simulink model "fft_biplex_test3"  (Simulink 7.6)
settings: Solver=ode45  StartTime=0.0  StopTime=5000  RelTol=1e-3
libraries: xbsIndex_r4 x1382, casper_library x82, monroe_library x27, xps_library x17, dspsigops x16, simulink x1
(part 9 of 13)

== system fft_biplex_test3/fft_biplex_real_4x1/biplex_core/fft_stage_2/delay_f ==
  In1 : Inport
  Constant2 : xbsIndex_r4/Constant  arith_type=Boolean  const=1  n_bits=1  bin_pt=0  explicit_period=on  period=1  equ=P=C  opselect=C  inp2=PCIN>>17  opr=+  inp1=P  carry=CIN  dbl_ovrd=off  block_type=constant
      settings: block_version=9.1.01
  Counter : xbsIndex_r4/Counter  cnt_type=Count Limited  cnt_to=DelayLen - bram_latency - 1  operation=Up  start_count=0  cnt_by_val=1  arith_type=Unsigned  n_bits=BitWidth  bin_pt=0  load_pin=off  rst=off  en=off  explicit_period=on  period=1  dbl_ovrd=off  use_behavioral_HDL=off  implementation=Fabric  use_rpm=off  block_type=counter
      settings: xl_area=[0, 0, 0, 0, 0, 0, 0]  block_version=9.1.01
  Single Port RAM : xbsIndex_r4/Single Port RAM  depth=2^BitWidth  initVector=0  distributed_mem=Block RAM  write_mode=Read Before Write  rst=off  init_reg=0  en=off  latency=bram_latency  dbl_ovrd=off  optimize=Area  use_rpm=off  block_type=spram
      settings: xl_area=[0, 0, 0, 0, 0, 0, 0]  block_version=9.1.01
  Out1 : Outport
  wires:
  Single Port RAM/1 -> Out1/1
  Counter/1 -> Single Port RAM/1
  In1/1 -> Single Port RAM/2
  Constant2/1 -> Single Port RAM/3

== system fft_biplex_test3/fft_biplex_real_4x1/biplex_core/fft_stage_3/butterfly_direct ==
  a : Inport
  b : Inport  Port=2
  sync : Inport  Port=3
  shift : Inport  Port=4
  Delay : xbsIndex_r4/Delay  en=off  latency=add_latency + 1  dbl_ovrd=off  reg_retiming=off  block_type=delay
      settings: xl_area=[0, 0, 0, 0, 0, 0, 0]  block_version=9.1.01
  Logical : xbsIndex_r4/Logical  logical_function=OR  inputs=4  en=off  latency=0  precision=Full  arith_type=Unsigned  n_bits=16  bin_pt=0  align_bp=on  dbl_ovrd=off  block_type=logical
      settings: block_version=10.1.1
  Register{,1..5} (6 alike) : xbsIndex_r4/Register  init=0  rst=off  en=off  dbl_ovrd=off  block_type=register
      settings: block_version=11.4
  Scale{,1..3} (4 alike) : xbsIndex_r4/Scale  scale_factor=-shift  dbl_ovrd=off  block_type=scale
      settings: block_version=9.1.01
  Terminator : Terminator
  convert_of1 : Subsystem  AncestorBlock=casper_library/Misc/convert_of  mask(convert_of){bit_width_i=24, binary_point_i=19, bit_width_o=18, binary_point_o=17, latency=1, overflow=Wrap, quantization=Truncate}
      mask prompts: bit_width_i "Bit Width In"; binary_point_i "Binary Point In"; bit_width_o "Bit Width Out"; binary_point_o "Binary Point Out"; overflow "Overflow Behaviour"; quantization "Quantization Behaviour"
      mask help:
      | Converts from one 2's complement bit-width
      | and/or binary point position to another.
      | Includes underflow/overflow indicator.
      mask init: same as fft_biplex_test3/fft_biplex_real_4x1/biplex_core/fft_stage_1/butterfly_direct/convert_of1
      settings: AttributesFormatString=[24,19]->[18,17]
      mask StyleString: edit,edit,edit,edit,edit,popup(Wrap|Saturate|Error),popup(Truncate|Round  (unbiased: +/- Inf)|Round  (unbiased: even values))
  convert_of2 : Subsystem  AncestorBlock=casper_library/FFTs/butterfly_direct/convert_of1  mask(convert_of){bit_width_i=24, binary_point_i=19, bit_width_o=18, binary_point_o=17, latency=1, overflow=Wrap, quantization=Truncate}
      mask prompts: bit_width_i "Bit Width In"; binary_point_i "Binary Point In"; bit_width_o "Bit Width Out"; binary_point_o "Binary Point Out"; overflow "Overflow Behaviour"; quantization "Quantization Behaviour"
      mask help:
      | Converts from one 2's complement bit-width
      | and/or binary point position to another.
      | Includes underflow/overflow indicator.
      mask init: same as fft_biplex_test3/fft_biplex_real_4x1/biplex_core/fft_stage_1/butterfly_direct/convert_of1
      settings: AttributesFormatString=[24,19]->[18,17]
      mask StyleString: edit,edit,edit,edit,edit,popup(Wrap|Saturate|Error),popup(Truncate|Round  (unbiased: +/- Inf)|Round  (unbiased: even values))
  convert_of3 : Subsystem  AncestorBlock=casper_library/FFTs/butterfly_direct/convert_of1  mask(convert_of){bit_width_i=24, binary_point_i=19, bit_width_o=18, binary_point_o=17, latency=1, overflow=Wrap, quantization=Truncate}
      mask prompts: bit_width_i "Bit Width In"; binary_point_i "Binary Point In"; bit_width_o "Bit Width Out"; binary_point_o "Binary Point Out"; overflow "Overflow Behaviour"; quantization "Quantization Behaviour"
      mask help:
      | Converts from one 2's complement bit-width
      | and/or binary point position to another.
      | Includes underflow/overflow indicator.
      mask init: same as fft_biplex_test3/fft_biplex_real_4x1/biplex_core/fft_stage_1/butterfly_direct/convert_of1
      settings: AttributesFormatString=[24,19]->[18,17]
      mask StyleString: edit,edit,edit,edit,edit,popup(Wrap|Saturate|Error),popup(Truncate|Round  (unbiased: +/- Inf)|Round  (unbiased: even values))
  convert_of4 : Subsystem  AncestorBlock=casper_library/FFTs/butterfly_direct/convert_of1  mask(convert_of){bit_width_i=24, binary_point_i=19, bit_width_o=18, binary_point_o=17, latency=1, overflow=Wrap, quantization=Truncate}
      mask prompts: bit_width_i "Bit Width In"; binary_point_i "Binary Point In"; bit_width_o "Bit Width Out"; binary_point_o "Binary Point Out"; overflow "Overflow Behaviour"; quantization "Quantization Behaviour"
      mask help:
      | Converts from one 2's complement bit-width
      | and/or binary point position to another.
      | Includes underflow/overflow indicator.
      mask init: same as fft_biplex_test3/fft_biplex_real_4x1/biplex_core/fft_stage_1/butterfly_direct/convert_of1
      settings: AttributesFormatString=[24,19]->[18,17]
      mask StyleString: edit,edit,edit,edit,edit,popup(Wrap|Saturate|Error),popup(Truncate|Round  (unbiased: +/- Inf)|Round  (unbiased: even values))
  dsp48_complex_add : Subsystem  mask{a_bit_width=18, a_bin_pt=17, bw_bit_width=input_bit_width+coeff_bit_width+1, bw_bin_pt=(input_bit_width - 1) + (coeff_bit_width-1)}
      mask prompts: a_bit_width "'a' bit width"; a_bin_pt "'a' binary point"; bw_bit_width "'bw' bit width"; bw_bin_pt "'bw' binary point"
  ri_to_c : casper_library/Misc/ri_to_c  SystemSampleTime=-1
  ri_to_c1 : casper_library/Misc/ri_to_c  SystemSampleTime=-1
  twiddle : Subsystem  AncestorBlock=casper_library/FFTs/Twiddle/twiddle_general_dsp48  mask(twiddle_general_dsp48){Coeffs=getfield( getfield( get_param( gcb,'UserData' ), 'parameters'),'Coeffs'), StepPeriod=2, coeffs_bram=off, coeff_bit_width=18, input_bit_width=18, add_latency=2, mult_latency=3, bram_latency=3, arch=Virtex5, use_hdl=on, use_embedded=off, quantization=Truncate, overflow=Wrap}
      mask prompts: Coeffs "Coefficients:"; StepPeriod "Coefficient Step Period (2^?)"; coeffs_bram "Store coefficients in BRAM"; coeff_bit_width "Coefficient Bit Width"; input_bit_width "Input Bit Width"; add_latency "Add Latency"; mult_latency "Mult Latency"; bram_latency "BRAM Latency"; arch "Architecture"; use_hdl "Use behavioural HDL for multipliers"; use_embedded "Use embedded multipliers"; quantization "Quantization Behavior"; overflow "Overflow Behavior"
      mask help:
      | Used in biplex pipelined FFT. Implements
      | (a+bi)(c+di) as (ac-bd)+i(ad+bc) with four
      | multipliers, manually instantiating dsp48 slices
      mask init:
      | twiddle_general_dsp48_init(gcb, ...
      |     'Coeffs', Coeffs, ...
      |     'StepPeriod', StepPeriod, ...
      |     'coeffs_bram', coeffs_bram, ...
      |     'coeff_bit_width', coeff_bit_width, ...
      |     'input_bit_width', input_bit_width, ...
      |     'add_latency', add_latency, ...
      |     'mult_latency', mult_latency, ...
      |     'bram_latency', bram_latency, ...
      |     'arch', arch, ...
      |     'use_hdl', use_hdl, ...
      |     'use_embedded', use_embedded, ...
      |     'quantization', quantization, ...
      |     'overflow', overflow)
      settings: AttributesFormatString=|
      | arch=Virtex5,
      |  input_bit_width=18,
      |  coeff_bit_width=18
      mask StyleString: edit,edit,checkbox,edit,edit,edit,edit,edit,popup(Virtex2Pro|Virtex5),checkbox,checkbox,popup(Truncate|Round  (unbiased: +/- Inf)|Round  (unbiased: Even Values)),popup(Wrap|Saturate|Error)
      mask CallbackString:
      | |||||||||use_hdl = get_param(gcb,'use_hdl');
      | visibs = get_param(gcb, 'MaskVisibilities');
      | if( strcmp(use_hdl,'on')),
      |     set_param(gcb, 'use_embedded','off');
      |     visibs{11} = 'off';
      | else,
      |     visibs{11} = 'on';
      | end
      | set_param(gcb, 'MaskVisibilities', visibs);|||
  a+bw : Outport
  a-bw : Outport  Port=2
  of : Outport  Port=3
  sync_out : Outport  Port=4
  wires:
  Register5/1 -> twiddle/1(a)
  Register4/1 -> twiddle/2(b)
  Register3/1 -> twiddle/3(sync)
  Register2/1 -> sync_out/1
  Register1/1 -> a-bw/1
  Register/1 -> a+bw/1
  dsp48_complex_add/4(a-bw_im) -> Scale3/1
  Logical/1 -> of/1
  shift/1 -> Terminator/1
  dsp48_complex_add/1(a+bw_re) -> Scale/1
  Delay/1 -> Register2/1
  ri_to_c1/1 -> Register1/1
  ri_to_c/1 -> Register/1
  a/1 -> Register5/1
  b/1 -> Register4/1
  sync/1 -> Register3/1
  twiddle/1(a_re) -> dsp48_complex_add/1(a_re)
  twiddle/2(a_im) -> dsp48_complex_add/2(a_im)
  twiddle/3(bw_re) -> dsp48_complex_add/3(bw_re)
  twiddle/4(bw_im) -> dsp48_complex_add/4(bw_im)
  twiddle/5(sync_out) -> Delay/1
  Scale/1 -> convert_of1/1(din)
  convert_of1/1(dout) -> ri_to_c/1
  dsp48_complex_add/2(a+bw_im) -> Scale1/1
  Scale1/1 -> convert_of2/1(din)
  convert_of2/1(dout) -> ri_to_c/2
  dsp48_complex_add/3(a-bw_re) -> Scale2/1
  Scale2/1 -> convert_of3/1(din)
  convert_of3/1(dout) -> ri_to_c1/1
  Scale3/1 -> convert_of4/1(din)
  convert_of4/1(dout) -> ri_to_c1/2
  convert_of1/2(of) -> Logical/1
  convert_of2/2(of) -> Logical/2
  convert_of3/2(of) -> Logical/3
  convert_of4/2(of) -> Logical/4

== system fft_biplex_test3/fft_biplex_real_4x1/biplex_core/fft_stage_3/delay_b ==
  In1 : Inport
  delay_slr : xbsIndex_r4/Delay  en=off  latency=DelayLen  dbl_ovrd=off  reg_retiming=off  block_type=delay
      settings: xl_area=[0, 0, 0, 0, 0, 0, 0]  block_version=9.1.01
  Out1 : Outport
  wires:
  In1/1 -> delay_slr/1
  delay_slr/1 -> Out1/1

== system fft_biplex_test3/fft_biplex_real_4x1/biplex_core/fft_stage_3/delay_f ==
  In1 : Inport
  delay_slr : xbsIndex_r4/Delay  en=off  latency=DelayLen  dbl_ovrd=off  reg_retiming=off  block_type=delay
      settings: xl_area=[0, 0, 0, 0, 0, 0, 0]  block_version=9.1.01
  Out1 : Outport
  wires:
  In1/1 -> delay_slr/1
  delay_slr/1 -> Out1/1

== system fft_biplex_test3/fft_biplex_real_4x1/biplex_core/fft_stage_4/butterfly_direct ==
  a : Inport
  b : Inport  Port=2
  sync : Inport  Port=3
  shift : Inport  Port=4
  Delay : xbsIndex_r4/Delay  en=off  latency=add_latency + 1  dbl_ovrd=off  reg_retiming=off  block_type=delay
      settings: xl_area=[0, 0, 0, 0, 0, 0, 0]  block_version=9.1.01
  Logical : xbsIndex_r4/Logical  logical_function=OR  inputs=4  en=off  latency=0  precision=Full  arith_type=Unsigned  n_bits=16  bin_pt=0  align_bp=on  dbl_ovrd=off  block_type=logical
      settings: block_version=10.1.1
  Register{,1..5} (6 alike) : xbsIndex_r4/Register  init=0  rst=off  en=off  dbl_ovrd=off  block_type=register
      settings: block_version=11.4
  Scale{,1..3} (4 alike) : xbsIndex_r4/Scale  scale_factor=-shift  dbl_ovrd=off  block_type=scale
      settings: block_version=9.1.01
  Terminator : Terminator
  convert_of1 : Subsystem  AncestorBlock=casper_library/Misc/convert_of  mask(convert_of){bit_width_i=24, binary_point_i=19, bit_width_o=18, binary_point_o=17, latency=1, overflow=Wrap, quantization=Truncate}
      mask prompts: bit_width_i "Bit Width In"; binary_point_i "Binary Point In"; bit_width_o "Bit Width Out"; binary_point_o "Binary Point Out"; overflow "Overflow Behaviour"; quantization "Quantization Behaviour"
      mask help:
      | Converts from one 2's complement bit-width
      | and/or binary point position to another.
      | Includes underflow/overflow indicator.
      mask init: same as fft_biplex_test3/fft_biplex_real_4x1/biplex_core/fft_stage_1/butterfly_direct/convert_of1
      settings: AttributesFormatString=[24,19]->[18,17]
      mask StyleString: edit,edit,edit,edit,edit,popup(Wrap|Saturate|Error),popup(Truncate|Round  (unbiased: +/- Inf)|Round  (unbiased: even values))
  convert_of2 : Subsystem  AncestorBlock=casper_library/FFTs/butterfly_direct/convert_of1  mask(convert_of){bit_width_i=24, binary_point_i=19, bit_width_o=18, binary_point_o=17, latency=1, overflow=Wrap, quantization=Truncate}
      mask prompts: bit_width_i "Bit Width In"; binary_point_i "Binary Point In"; bit_width_o "Bit Width Out"; binary_point_o "Binary Point Out"; overflow "Overflow Behaviour"; quantization "Quantization Behaviour"
      mask help:
      | Converts from one 2's complement bit-width
      | and/or binary point position to another.
      | Includes underflow/overflow indicator.
      mask init: same as fft_biplex_test3/fft_biplex_real_4x1/biplex_core/fft_stage_1/butterfly_direct/convert_of1
      settings: AttributesFormatString=[24,19]->[18,17]
      mask StyleString: edit,edit,edit,edit,edit,popup(Wrap|Saturate|Error),popup(Truncate|Round  (unbiased: +/- Inf)|Round  (unbiased: even values))
  convert_of3 : Subsystem  AncestorBlock=casper_library/FFTs/butterfly_direct/convert_of1  mask(convert_of){bit_width_i=24, binary_point_i=19, bit_width_o=18, binary_point_o=17, latency=1, overflow=Wrap, quantization=Truncate}
      mask prompts: bit_width_i "Bit Width In"; binary_point_i "Binary Point In"; bit_width_o "Bit Width Out"; binary_point_o "Binary Point Out"; overflow "Overflow Behaviour"; quantization "Quantization Behaviour"
      mask help:
      | Converts from one 2's complement bit-width
      | and/or binary point position to another.
      | Includes underflow/overflow indicator.
      mask init: same as fft_biplex_test3/fft_biplex_real_4x1/biplex_core/fft_stage_1/butterfly_direct/convert_of1
      settings: AttributesFormatString=[24,19]->[18,17]
      mask StyleString: edit,edit,edit,edit,edit,popup(Wrap|Saturate|Error),popup(Truncate|Round  (unbiased: +/- Inf)|Round  (unbiased: even values))
  convert_of4 : Subsystem  AncestorBlock=casper_library/FFTs/butterfly_direct/convert_of1  mask(convert_of){bit_width_i=24, binary_point_i=19, bit_width_o=18, binary_point_o=17, latency=1, overflow=Wrap, quantization=Truncate}
      mask prompts: bit_width_i "Bit Width In"; binary_point_i "Binary Point In"; bit_width_o "Bit Width Out"; binary_point_o "Binary Point Out"; overflow "Overflow Behaviour"; quantization "Quantization Behaviour"
      mask help:
      | Converts from one 2's complement bit-width
      | and/or binary point position to another.
      | Includes underflow/overflow indicator.
      mask init: same as fft_biplex_test3/fft_biplex_real_4x1/biplex_core/fft_stage_1/butterfly_direct/convert_of1
      settings: AttributesFormatString=[24,19]->[18,17]
      mask StyleString: edit,edit,edit,edit,edit,popup(Wrap|Saturate|Error),popup(Truncate|Round  (unbiased: +/- Inf)|Round  (unbiased: even values))
  dsp48_complex_add : Subsystem  mask{a_bit_width=18, a_bin_pt=17, bw_bit_width=input_bit_width+coeff_bit_width+1, bw_bin_pt=(input_bit_width - 1) + (coeff_bit_width-1)}
      mask prompts: a_bit_width "'a' bit width"; a_bin_pt "'a' binary point"; bw_bit_width "'bw' bit width"; bw_bin_pt "'bw' binary point"
  ri_to_c : casper_library/Misc/ri_to_c  SystemSampleTime=-1
  ri_to_c1 : casper_library/Misc/ri_to_c  SystemSampleTime=-1
  twiddle : Subsystem  AncestorBlock=casper_library/FFTs/Twiddle/twiddle_general_dsp48  mask(twiddle_general_dsp48){Coeffs=getfield( getfield( get_param( gcb,'UserData' ), 'parameters'),'Coeffs'), StepPeriod=1, coeffs_bram=off, coeff_bit_width=18, input_bit_width=18, add_latency=2, mult_latency=3, bram_latency=3, arch=Virtex5, use_hdl=on, use_embedded=off, quantization=Truncate, overflow=Wrap}
      mask prompts: Coeffs "Coefficients:"; StepPeriod "Coefficient Step Period (2^?)"; coeffs_bram "Store coefficients in BRAM"; coeff_bit_width "Coefficient Bit Width"; input_bit_width "Input Bit Width"; add_latency "Add Latency"; mult_latency "Mult Latency"; bram_latency "BRAM Latency"; arch "Architecture"; use_hdl "Use behavioural HDL for multipliers"; use_embedded "Use embedded multipliers"; quantization "Quantization Behavior"; overflow "Overflow Behavior"
      mask help:
      | Used in biplex pipelined FFT. Implements
      | (a+bi)(c+di) as (ac-bd)+i(ad+bc) with four
      | multipliers, manually instantiating dsp48 slices
      mask init: same as fft_biplex_test3/fft_biplex_real_4x1/biplex_core/fft_stage_3/butterfly_direct/twiddle
      settings: AttributesFormatString=|
      | arch=Virtex5,
      |  input_bit_width=18,
      |  coeff_bit_width=18
      mask StyleString: edit,edit,checkbox,edit,edit,edit,edit,edit,popup(Virtex2Pro|Virtex5),checkbox,checkbox,popup(Truncate|Round  (unbiased: +/- Inf)|Round  (unbiased: Even Values)),popup(Wrap|Saturate|Error)
      mask CallbackString:
      | |||||||||use_hdl = get_param(gcb,'use_hdl');
      | visibs = get_param(gcb, 'MaskVisibilities');
      | if( strcmp(use_hdl,'on')),
      |     set_param(gcb, 'use_embedded','off');
      |     visibs{11} = 'off';
      | else,
      |     visibs{11} = 'on';
      | end
      | set_param(gcb, 'MaskVisibilities', visibs);|||
  a+bw : Outport
  a-bw : Outport  Port=2
  of : Outport  Port=3
  sync_out : Outport  Port=4
  wires:
  Register5/1 -> twiddle/1(a)
  Register4/1 -> twiddle/2(b)
  Register3/1 -> twiddle/3(sync)
  Register2/1 -> sync_out/1
  Register1/1 -> a-bw/1
  Register/1 -> a+bw/1
  dsp48_complex_add/4(a-bw_im) -> Scale3/1
  Logical/1 -> of/1
  shift/1 -> Terminator/1
  dsp48_complex_add/1(a+bw_re) -> Scale/1
  Delay/1 -> Register2/1
  ri_to_c1/1 -> Register1/1
  ri_to_c/1 -> Register/1
  a/1 -> Register5/1
  b/1 -> Register4/1
  sync/1 -> Register3/1
  twiddle/1(a_re) -> dsp48_complex_add/1(a_re)
  twiddle/2(a_im) -> dsp48_complex_add/2(a_im)
  twiddle/3(bw_re) -> dsp48_complex_add/3(bw_re)
  twiddle/4(bw_im) -> dsp48_complex_add/4(bw_im)
  twiddle/5(sync_out) -> Delay/1
  Scale/1 -> convert_of1/1(din)
  convert_of1/1(dout) -> ri_to_c/1
  dsp48_complex_add/2(a+bw_im) -> Scale1/1
  Scale1/1 -> convert_of2/1(din)
  convert_of2/1(dout) -> ri_to_c/2
  dsp48_complex_add/3(a-bw_re) -> Scale2/1
  Scale2/1 -> convert_of3/1(din)
  convert_of3/1(dout) -> ri_to_c1/1
  Scale3/1 -> convert_of4/1(din)
  convert_of4/1(dout) -> ri_to_c1/2
  convert_of1/2(of) -> Logical/1
  convert_of2/2(of) -> Logical/2
  convert_of3/2(of) -> Logical/3
  convert_of4/2(of) -> Logical/4

== system fft_biplex_test3/fft_biplex_real_4x1/biplex_core/fft_stage_4/delay_b ==
  In1 : Inport
  delay_slr : xbsIndex_r4/Delay  en=off  latency=DelayLen  dbl_ovrd=off  reg_retiming=off  block_type=delay
      settings: xl_area=[0, 0, 0, 0, 0, 0, 0]  block_version=9.1.01
  Out1 : Outport
  wires:
  In1/1 -> delay_slr/1
  delay_slr/1 -> Out1/1

== system fft_biplex_test3/fft_biplex_real_4x1/biplex_core/fft_stage_4/delay_f ==
  In1 : Inport
  delay_slr : xbsIndex_r4/Delay  en=off  latency=DelayLen  dbl_ovrd=off  reg_retiming=off  block_type=delay
      settings: xl_area=[0, 0, 0, 0, 0, 0, 0]  block_version=9.1.01
  Out1 : Outport
  wires:
  In1/1 -> delay_slr/1
  delay_slr/1 -> Out1/1

== system fft_biplex_test3/fft_biplex_real_4x1/biplex_core/fft_stage_5/butterfly_direct ==
  a : Inport
  b : Inport  Port=2
  sync : Inport  Port=3
  shift : Inport  Port=4
  Delay : xbsIndex_r4/Delay  en=off  latency=add_latency + 1  dbl_ovrd=off  reg_retiming=off  block_type=delay
      settings: xl_area=[0, 0, 0, 0, 0, 0, 0]  block_version=9.1.01
  Logical : xbsIndex_r4/Logical  logical_function=OR  inputs=4  en=off  latency=0  precision=Full  arith_type=Unsigned  n_bits=16  bin_pt=0  align_bp=on  dbl_ovrd=off  block_type=logical
      settings: block_version=10.1.1
  Register{,1..5} (6 alike) : xbsIndex_r4/Register  init=0  rst=off  en=off  dbl_ovrd=off  block_type=register
      settings: block_version=11.4
  Scale{,1..3} (4 alike) : xbsIndex_r4/Scale  scale_factor=-shift  dbl_ovrd=off  block_type=scale
      settings: block_version=9.1.01
  Terminator : Terminator
  convert_of1 : Subsystem  AncestorBlock=casper_library/Misc/convert_of  mask(convert_of){bit_width_i=24, binary_point_i=19, bit_width_o=18, binary_point_o=17, latency=1, overflow=Wrap, quantization=Truncate}
      mask prompts: bit_width_i "Bit Width In"; binary_point_i "Binary Point In"; bit_width_o "Bit Width Out"; binary_point_o "Binary Point Out"; overflow "Overflow Behaviour"; quantization "Quantization Behaviour"
      mask help:
      | Converts from one 2's complement bit-width
      | and/or binary point position to another.
      | Includes underflow/overflow indicator.
      mask init: same as fft_biplex_test3/fft_biplex_real_4x1/biplex_core/fft_stage_1/butterfly_direct/convert_of1
      settings: AttributesFormatString=[24,19]->[18,17]
      mask StyleString: edit,edit,edit,edit,edit,popup(Wrap|Saturate|Error),popup(Truncate|Round  (unbiased: +/- Inf)|Round  (unbiased: even values))
  convert_of2 : Subsystem  AncestorBlock=casper_library/FFTs/butterfly_direct/convert_of1  mask(convert_of){bit_width_i=24, binary_point_i=19, bit_width_o=18, binary_point_o=17, latency=1, overflow=Wrap, quantization=Truncate}
      mask prompts: bit_width_i "Bit Width In"; binary_point_i "Binary Point In"; bit_width_o "Bit Width Out"; binary_point_o "Binary Point Out"; overflow "Overflow Behaviour"; quantization "Quantization Behaviour"
      mask help:
      | Converts from one 2's complement bit-width
      | and/or binary point position to another.
      | Includes underflow/overflow indicator.
      mask init: same as fft_biplex_test3/fft_biplex_real_4x1/biplex_core/fft_stage_1/butterfly_direct/convert_of1
      settings: AttributesFormatString=[24,19]->[18,17]
      mask StyleString: edit,edit,edit,edit,edit,popup(Wrap|Saturate|Error),popup(Truncate|Round  (unbiased: +/- Inf)|Round  (unbiased: even values))
  convert_of3 : Subsystem  AncestorBlock=casper_library/FFTs/butterfly_direct/convert_of1  mask(convert_of){bit_width_i=24, binary_point_i=19, bit_width_o=18, binary_point_o=17, latency=1, overflow=Wrap, quantization=Truncate}
      mask prompts: bit_width_i "Bit Width In"; binary_point_i "Binary Point In"; bit_width_o "Bit Width Out"; binary_point_o "Binary Point Out"; overflow "Overflow Behaviour"; quantization "Quantization Behaviour"
      mask help:
      | Converts from one 2's complement bit-width
      | and/or binary point position to another.
      | Includes underflow/overflow indicator.
      mask init: same as fft_biplex_test3/fft_biplex_real_4x1/biplex_core/fft_stage_1/butterfly_direct/convert_of1
      settings: AttributesFormatString=[24,19]->[18,17]
      mask StyleString: edit,edit,edit,edit,edit,popup(Wrap|Saturate|Error),popup(Truncate|Round  (unbiased: +/- Inf)|Round  (unbiased: even values))
  convert_of4 : Subsystem  AncestorBlock=casper_library/FFTs/butterfly_direct/convert_of1  mask(convert_of){bit_width_i=24, binary_point_i=19, bit_width_o=18, binary_point_o=17, latency=1, overflow=Wrap, quantization=Truncate}
      mask prompts: bit_width_i "Bit Width In"; binary_point_i "Binary Point In"; bit_width_o "Bit Width Out"; binary_point_o "Binary Point Out"; overflow "Overflow Behaviour"; quantization "Quantization Behaviour"
      mask help:
      | Converts from one 2's complement bit-width
      | and/or binary point position to another.
      | Includes underflow/overflow indicator.
      mask init: same as fft_biplex_test3/fft_biplex_real_4x1/biplex_core/fft_stage_1/butterfly_direct/convert_of1
      settings: AttributesFormatString=[24,19]->[18,17]
      mask StyleString: edit,edit,edit,edit,edit,popup(Wrap|Saturate|Error),popup(Truncate|Round  (unbiased: +/- Inf)|Round  (unbiased: even values))
  dsp48_complex_add : Subsystem  mask{a_bit_width=18, a_bin_pt=17, bw_bit_width=input_bit_width+coeff_bit_width+1, bw_bin_pt=(input_bit_width - 1) + (coeff_bit_width-1)}
      mask prompts: a_bit_width "'a' bit width"; a_bin_pt "'a' binary point"; bw_bit_width "'bw' bit width"; bw_bin_pt "'bw' binary point"
  ri_to_c : casper_library/Misc/ri_to_c  SystemSampleTime=-1
  ri_to_c1 : casper_library/Misc/ri_to_c  SystemSampleTime=-1
  twiddle : Subsystem  AncestorBlock=casper_library/FFTs/Twiddle/twiddle_general_dsp48  mask(twiddle_general_dsp48){Coeffs=getfield( getfield( get_param( gcb,'UserData' ), 'parameters'),'Coeffs'), StepPeriod=0, coeffs_bram=off, coeff_bit_width=18, input_bit_width=18, add_latency=2, mult_latency=3, bram_latency=3, arch=Virtex5, use_hdl=on, use_embedded=off, quantization=Truncate, overflow=Wrap}
      mask prompts: Coeffs "Coefficients:"; StepPeriod "Coefficient Step Period (2^?)"; coeffs_bram "Store coefficients in BRAM"; coeff_bit_width "Coefficient Bit Width"; input_bit_width "Input Bit Width"; add_latency "Add Latency"; mult_latency "Mult Latency"; bram_latency "BRAM Latency"; arch "Architecture"; use_hdl "Use behavioural HDL for multipliers"; use_embedded "Use embedded multipliers"; quantization "Quantization Behavior"; overflow "Overflow Behavior"
      mask help:
      | Used in biplex pipelined FFT. Implements
      | (a+bi)(c+di) as (ac-bd)+i(ad+bc) with four
      | multipliers, manually instantiating dsp48 slices
      mask init: same as fft_biplex_test3/fft_biplex_real_4x1/biplex_core/fft_stage_3/butterfly_direct/twiddle
      settings: AttributesFormatString=|
      | arch=Virtex5,
      |  input_bit_width=18,
      |  coeff_bit_width=18
      mask StyleString: edit,edit,checkbox,edit,edit,edit,edit,edit,popup(Virtex2Pro|Virtex5),checkbox,checkbox,popup(Truncate|Round  (unbiased: +/- Inf)|Round  (unbiased: Even Values)),popup(Wrap|Saturate|Error)
      mask CallbackString:
      | |||||||||use_hdl = get_param(gcb,'use_hdl');
      | visibs = get_param(gcb, 'MaskVisibilities');
      | if( strcmp(use_hdl,'on')),
      |     set_param(gcb, 'use_embedded','off');
      |     visibs{11} = 'off';
      | else,
      |     visibs{11} = 'on';
      | end
      | set_param(gcb, 'MaskVisibilities', visibs);|||
  a+bw : Outport
  a-bw : Outport  Port=2
  of : Outport  Port=3
  sync_out : Outport  Port=4
  wires:
  Register5/1 -> twiddle/1(a)
  Register4/1 -> twiddle/2(b)
  Register3/1 -> twiddle/3(sync)
  Register2/1 -> sync_out/1
  Register1/1 -> a-bw/1
  Register/1 -> a+bw/1
  dsp48_complex_add/4(a-bw_im) -> Scale3/1
  Logical/1 -> of/1
  shift/1 -> Terminator/1
  dsp48_complex_add/1(a+bw_re) -> Scale/1
  Delay/1 -> Register2/1
  ri_to_c1/1 -> Register1/1
  ri_to_c/1 -> Register/1
  a/1 -> Register5/1
  b/1 -> Register4/1
  sync/1 -> Register3/1
  twiddle/1(a_re) -> dsp48_complex_add/1(a_re)
  twiddle/2(a_im) -> dsp48_complex_add/2(a_im)
  twiddle/3(bw_re) -> dsp48_complex_add/3(bw_re)
  twiddle/4(bw_im) -> dsp48_complex_add/4(bw_im)
  twiddle/5(sync_out) -> Delay/1
  Scale/1 -> convert_of1/1(din)
  convert_of1/1(dout) -> ri_to_c/1
  dsp48_complex_add/2(a+bw_im) -> Scale1/1
  Scale1/1 -> convert_of2/1(din)
  convert_of2/1(dout) -> ri_to_c/2
  dsp48_complex_add/3(a-bw_re) -> Scale2/1
  Scale2/1 -> convert_of3/1(din)
  convert_of3/1(dout) -> ri_to_c1/1
  Scale3/1 -> convert_of4/1(din)
  convert_of4/1(dout) -> ri_to_c1/2
  convert_of1/2(of) -> Logical/1
  convert_of2/2(of) -> Logical/2
  convert_of3/2(of) -> Logical/3
  convert_of4/2(of) -> Logical/4

== system fft_biplex_test3/fft_biplex_real_4x1/biplex_core/fft_stage_5/delay_b ==
  In1 : Inport
  delay_slr : xbsIndex_r4/Delay  en=off  latency=DelayLen  dbl_ovrd=off  reg_retiming=off  block_type=delay
      settings: xl_area=[0, 0, 0, 0, 0, 0, 0]  block_version=9.1.01
  Out1 : Outport
  wires:
  In1/1 -> delay_slr/1
  delay_slr/1 -> Out1/1

== system fft_biplex_test3/fft_biplex_real_4x1/biplex_core/fft_stage_5/delay_f ==
  In1 : Inport
  delay_slr : xbsIndex_r4/Delay  en=off  latency=DelayLen  dbl_ovrd=off  reg_retiming=off  block_type=delay
      settings: xl_area=[0, 0, 0, 0, 0, 0, 0]  block_version=9.1.01
  Out1 : Outport
  wires:
  In1/1 -> delay_slr/1
  delay_slr/1 -> Out1/1

== system fft_biplex_test3/fft_biplex_real_4x1/bi_real_unscr_4x/mirror_spectrum/complex_conj/negate_dsp48 ==
  In1 : Inport
  Convert : xbsIndex_r4/Convert  arith_type="Signed  (2's comp)"  n_bits=18  bin_pt=input_bin_pt  quantization=Truncate  overflow=Wrap  en=off  latency=0  dbl_ovrd=off  pipeline=off  block_type=convert
      settings: block_version=11.4
  Convert1 : xbsIndex_r4/Convert  arith_type="Signed  (2's comp)"  n_bits=input_bit_width  bin_pt=input_bin_pt  quantization=Truncate  overflow=Wrap  en=off  latency=0  dbl_ovrd=off  pipeline=off  block_type=convert
      settings: block_version=11.4
  Reinterpret : xbsIndex_r4/Reinterpret  force_arith_type=on  arith_type="Signed  (2's comp)"  force_bin_pt=on  bin_pt=input_bin_pt  block_type=reinterpret
      settings: infoedit="Changes signal type without altering the binary representation.   You can changed the signal between signed and unsigned, and relocate the binary point.<br><br>Hardware notes: In hardware this block costs nothing.<br><br>Example:  Suppose the input is 6 bits wide, signed, with 2 fractional bits, and the output is forced to unsigned with 0 fractional bits.  Then an input of -2.0 (1110.00 in binary 2's complement) becomes an output of 56 (111000 in binary)."
  Reinterpret1 : xbsIndex_r4/Reinterpret  force_arith_type=on  arith_type="Signed  (2's comp)"  force_bin_pt=on  bin_pt=0  block_type=reinterpret
      settings: infoedit="Changes signal type without altering the binary representation.   You can changed the signal between signed and unsigned, and relocate the binary point.<br><br>Hardware notes: In hardware this block costs nothing.<br><br>Example:  Suppose the input is 6 bits wide, signed, with 2 fractional bits, and the output is forced to unsigned with 0 fractional bits.  Then an input of -2.0 (1110.00 in binary 2's complement) becomes an output of 56 (111000 in binary)."
  alucode3 : xbsIndex_r4/Constant  arith_type=Unsigned  const=0  n_bits=4  bin_pt=0  explicit_period=on  period=1  equ=P=C  opselect=C  inp2=PCIN>>17  opr=+  inp1=P  carry=CIN  dbl_ovrd=off  block_type=constant
  carryin3 : xbsIndex_r4/Constant  arith_type=Unsigned  const=0  n_bits=1  bin_pt=0  explicit_period=on  period=1  equ=P=C  opselect=C  inp2=PCIN>>17  opr=+  inp1=P  carry=CIN  dbl_ovrd=off  block_type=constant
  carryinsel3 : xbsIndex_r4/Constant  arith_type=Unsigned  const=0  n_bits=3  bin_pt=0  explicit_period=on  period=1  equ=P=C  opselect=C  inp2=PCIN>>17  opr=+  inp1=P  carry=CIN  dbl_ovrd=off  block_type=constant
  negate_dsp48 : xbsIndex_r4/DSP48E  use_a=Direct from A Port  use_b=Direct from B Port  reset_preg=off  pattern_from_creg=off  pattern='000000000000'  mask_from_creg=off  pattern_mask='3FFFFFFFFFFF'  sel_rounding_mask=Select mask  use_op=off  use_creg=off  rst_all=off  en_all=off  use_pcin=off  use_carrycascin=off  use_multsignin=off  use_carryout=off  use_patterndetect=off  use_patternbdetect=off  use_overflow=off  use_underflow=off  use_acout=off  use_bcout=off  use_pcout=off  use_multsignout=off  use_carrycascout=off  pipeline_a=1  pipeline_b=1  pipeline_acout=1  pipeline_bcout=1  pipeline_c=on  pipeline_p=on  pipeline_mult=on  pipeline_opmode=on  pipeline_alumode=on  pipeline_carryin=on  pipeline_carryinsel=on  rst_a=off  rst_b=off  rst_c=off  rst_mult=off  rst_p=off  rst_carry_in=off  rst_alumode=off  rst_ctrl=off  en_a1=off  en_a2=off  en_b1=off  en_b2=off  en_c=off  en_mult=off  en_p=off  en_carry_in=off  en_alumode=off  en_multcarryin=off  en_ctrl=off  use_synth_model=off  addsub_mode=ONE48  xl_useadderonly=off  block_type=dsp48e
      settings: block_version=10.1.3
  opcode1 : xbsIndex_r4/Constant  arith_type=Signed (2's comp)  const=-1  n_bits=30  bin_pt=0  explicit_period=on  period=1  equ=P=C  opselect=C  inp2=PCIN>>17  opr=+  inp1=P  carry=CIN  dbl_ovrd=off  block_type=constant
  opcode3 : xbsIndex_r4/Constant  arith_type=Unsigned  const=5  n_bits=7  bin_pt=0  explicit_period=on  period=1  equ=P=C  opselect=C  inp2=PCIN>>17  opr=+  inp1=P  carry=CIN  dbl_ovrd=off  block_type=constant
  Out1 : Outport
  wires:
  negate_dsp48/1 -> Reinterpret/1
  In1/1 -> Convert/1
  Reinterpret1/1 -> negate_dsp48/2
  Convert/1 -> Reinterpret1/1
  opcode1/1 -> negate_dsp48/1
  opcode3/1 -> negate_dsp48/3
  alucode3/1 -> negate_dsp48/4
  carryin3/1 -> negate_dsp48/5
  carryinsel3/1 -> negate_dsp48/6
  Reinterpret/1 -> Convert1/1
  Convert1/1 -> Out1/1

== system fft_biplex_test3/fft_biplex_real_4x1/bi_real_unscr_4x/mirror_spectrum/complex_conj1/negate_dsp48 ==
  In1 : Inport
  Convert : xbsIndex_r4/Convert  arith_type="Signed  (2's comp)"  n_bits=18  bin_pt=input_bin_pt  quantization=Truncate  overflow=Wrap  en=off  latency=0  dbl_ovrd=off  pipeline=off  block_type=convert
      settings: block_version=11.4
  Convert1 : xbsIndex_r4/Convert  arith_type="Signed  (2's comp)"  n_bits=input_bit_width  bin_pt=input_bin_pt  quantization=Truncate  overflow=Wrap  en=off  latency=0  dbl_ovrd=off  pipeline=off  block_type=convert
      settings: block_version=11.4
  Reinterpret : xbsIndex_r4/Reinterpret  force_arith_type=on  arith_type="Signed  (2's comp)"  force_bin_pt=on  bin_pt=input_bin_pt  block_type=reinterpret
      settings: infoedit="Changes signal type without altering the binary representation.   You can changed the signal between signed and unsigned, and relocate the binary point.<br><br>Hardware notes: In hardware this block costs nothing.<br><br>Example:  Suppose the input is 6 bits wide, signed, with 2 fractional bits, and the output is forced to unsigned with 0 fractional bits.  Then an input of -2.0 (1110.00 in binary 2's complement) becomes an output of 56 (111000 in binary)."
  Reinterpret1 : xbsIndex_r4/Reinterpret  force_arith_type=on  arith_type="Signed  (2's comp)"  force_bin_pt=on  bin_pt=0  block_type=reinterpret
      settings: infoedit="Changes signal type without altering the binary representation.   You can changed the signal between signed and unsigned, and relocate the binary point.<br><br>Hardware notes: In hardware this block costs nothing.<br><br>Example:  Suppose the input is 6 bits wide, signed, with 2 fractional bits, and the output is forced to unsigned with 0 fractional bits.  Then an input of -2.0 (1110.00 in binary 2's complement) becomes an output of 56 (111000 in binary)."
  alucode3 : xbsIndex_r4/Constant  arith_type=Unsigned  const=0  n_bits=4  bin_pt=0  explicit_period=on  period=1  equ=P=C  opselect=C  inp2=PCIN>>17  opr=+  inp1=P  carry=CIN  dbl_ovrd=off  block_type=constant
  carryin3 : xbsIndex_r4/Constant  arith_type=Unsigned  const=0  n_bits=1  bin_pt=0  explicit_period=on  period=1  equ=P=C  opselect=C  inp2=PCIN>>17  opr=+  inp1=P  carry=CIN  dbl_ovrd=off  block_type=constant
  carryinsel3 : xbsIndex_r4/Constant  arith_type=Unsigned  const=0  n_bits=3  bin_pt=0  explicit_period=on  period=1  equ=P=C  opselect=C  inp2=PCIN>>17  opr=+  inp1=P  carry=CIN  dbl_ovrd=off  block_type=constant
  negate_dsp48 : xbsIndex_r4/DSP48E  use_a=Direct from A Port  use_b=Direct from B Port  reset_preg=off  pattern_from_creg=off  pattern='000000000000'  mask_from_creg=off  pattern_mask='3FFFFFFFFFFF'  sel_rounding_mask=Select mask  use_op=off  use_creg=off  rst_all=off  en_all=off  use_pcin=off  use_carrycascin=off  use_multsignin=off  use_carryout=off  use_patterndetect=off  use_patternbdetect=off  use_overflow=off  use_underflow=off  use_acout=off  use_bcout=off  use_pcout=off  use_multsignout=off  use_carrycascout=off  pipeline_a=1  pipeline_b=1  pipeline_acout=1  pipeline_bcout=1  pipeline_c=on  pipeline_p=on  pipeline_mult=on  pipeline_opmode=on  pipeline_alumode=on  pipeline_carryin=on  pipeline_carryinsel=on  rst_a=off  rst_b=off  rst_c=off  rst_mult=off  rst_p=off  rst_carry_in=off  rst_alumode=off  rst_ctrl=off  en_a1=off  en_a2=off  en_b1=off  en_b2=off  en_c=off  en_mult=off  en_p=off  en_carry_in=off  en_alumode=off  en_multcarryin=off  en_ctrl=off  use_synth_model=off  addsub_mode=ONE48  xl_useadderonly=off  block_type=dsp48e
      settings: block_version=10.1.3
  opcode1 : xbsIndex_r4/Constant  arith_type=Signed (2's comp)  const=-1  n_bits=30  bin_pt=0  explicit_period=on  period=1  equ=P=C  opselect=C  inp2=PCIN>>17  opr=+  inp1=P  carry=CIN  dbl_ovrd=off  block_type=constant
  opcode3 : xbsIndex_r4/Constant  arith_type=Unsigned  const=5  n_bits=7  bin_pt=0  explicit_period=on  period=1  equ=P=C  opselect=C  inp2=PCIN>>17  opr=+  inp1=P  carry=CIN  dbl_ovrd=off  block_type=constant
  Out1 : Outport
  wires:
  Convert1/1 -> Out1/1
  Reinterpret/1 -> Convert1/1
  carryinsel3/1 -> negate_dsp48/6
  carryin3/1 -> negate_dsp48/5
  alucode3/1 -> negate_dsp48/4
  opcode3/1 -> negate_dsp48/3
  opcode1/1 -> negate_dsp48/1
  Convert/1 -> Reinterpret1/1
  Reinterpret1/1 -> negate_dsp48/2
  In1/1 -> Convert/1
  negate_dsp48/1 -> Reinterpret/1

== system fft_biplex_test3/fft_biplex_real_4x1/bi_real_unscr_4x/mirror_spectrum/complex_conj2/negate_dsp48 ==
  In1 : Inport
  Convert : xbsIndex_r4/Convert  arith_type="Signed  (2's comp)"  n_bits=18  bin_pt=input_bin_pt  quantization=Truncate  overflow=Wrap  en=off  latency=0  dbl_ovrd=off  pipeline=off  block_type=convert
      settings: block_version=11.4
  Convert1 : xbsIndex_r4/Convert  arith_type="Signed  (2's comp)"  n_bits=input_bit_width  bin_pt=input_bin_pt  quantization=Truncate  overflow=Wrap  en=off  latency=0  dbl_ovrd=off  pipeline=off  block_type=convert
      settings: block_version=11.4
  Reinterpret : xbsIndex_r4/Reinterpret  force_arith_type=on  arith_type="Signed  (2's comp)"  force_bin_pt=on  bin_pt=input_bin_pt  block_type=reinterpret
      settings: infoedit="Changes signal type without altering the binary representation.   You can changed the signal between signed and unsigned, and relocate the binary point.<br><br>Hardware notes: In hardware this block costs nothing.<br><br>Example:  Suppose the input is 6 bits wide, signed, with 2 fractional bits, and the output is forced to unsigned with 0 fractional bits.  Then an input of -2.0 (1110.00 in binary 2's complement) becomes an output of 56 (111000 in binary)."
  Reinterpret1 : xbsIndex_r4/Reinterpret  force_arith_type=on  arith_type="Signed  (2's comp)"  force_bin_pt=on  bin_pt=0  block_type=reinterpret
      settings: infoedit="Changes signal type without altering the binary representation.   You can changed the signal between signed and unsigned, and relocate the binary point.<br><br>Hardware notes: In hardware this block costs nothing.<br><br>Example:  Suppose the input is 6 bits wide, signed, with 2 fractional bits, and the output is forced to unsigned with 0 fractional bits.  Then an input of -2.0 (1110.00 in binary 2's complement) becomes an output of 56 (111000 in binary)."
  alucode3 : xbsIndex_r4/Constant  arith_type=Unsigned  const=0  n_bits=4  bin_pt=0  explicit_period=on  period=1  equ=P=C  opselect=C  inp2=PCIN>>17  opr=+  inp1=P  carry=CIN  dbl_ovrd=off  block_type=constant
  carryin3 : xbsIndex_r4/Constant  arith_type=Unsigned  const=0  n_bits=1  bin_pt=0  explicit_period=on  period=1  equ=P=C  opselect=C  inp2=PCIN>>17  opr=+  inp1=P  carry=CIN  dbl_ovrd=off  block_type=constant
  carryinsel3 : xbsIndex_r4/Constant  arith_type=Unsigned  const=0  n_bits=3  bin_pt=0  explicit_period=on  period=1  equ=P=C  opselect=C  inp2=PCIN>>17  opr=+  inp1=P  carry=CIN  dbl_ovrd=off  block_type=constant
  negate_dsp48 : xbsIndex_r4/DSP48E  use_a=Direct from A Port  use_b=Direct from B Port  reset_preg=off  pattern_from_creg=off  pattern='000000000000'  mask_from_creg=off  pattern_mask='3FFFFFFFFFFF'  sel_rounding_mask=Select mask  use_op=off  use_creg=off  rst_all=off  en_all=off  use_pcin=off  use_carrycascin=off  use_multsignin=off  use_carryout=off  use_patterndetect=off  use_patternbdetect=off  use_overflow=off  use_underflow=off  use_acout=off  use_bcout=off  use_pcout=off  use_multsignout=off  use_carrycascout=off  pipeline_a=1  pipeline_b=1  pipeline_acout=1  pipeline_bcout=1  pipeline_c=on  pipeline_p=on  pipeline_mult=on  pipeline_opmode=on  pipeline_alumode=on  pipeline_carryin=on  pipeline_carryinsel=on  rst_a=off  rst_b=off  rst_c=off  rst_mult=off  rst_p=off  rst_carry_in=off  rst_alumode=off  rst_ctrl=off  en_a1=off  en_a2=off  en_b1=off  en_b2=off  en_c=off  en_mult=off  en_p=off  en_carry_in=off  en_alumode=off  en_multcarryin=off  en_ctrl=off  use_synth_model=off  addsub_mode=ONE48  xl_useadderonly=off  block_type=dsp48e
      settings: block_version=10.1.3
  opcode1 : xbsIndex_r4/Constant  arith_type=Signed (2's comp)  const=-1  n_bits=30  bin_pt=0  explicit_period=on  period=1  equ=P=C  opselect=C  inp2=PCIN>>17  opr=+  inp1=P  carry=CIN  dbl_ovrd=off  block_type=constant
  opcode3 : xbsIndex_r4/Constant  arith_type=Unsigned  const=5  n_bits=7  bin_pt=0  explicit_period=on  period=1  equ=P=C  opselect=C  inp2=PCIN>>17  opr=+  inp1=P  carry=CIN  dbl_ovrd=off  block_type=constant
  Out1 : Outport
  wires:
  negate_dsp48/1 -> Reinterpret/1
  In1/1 -> Convert/1
  Reinterpret1/1 -> negate_dsp48/2
  Convert/1 -> Reinterpret1/1
  opcode1/1 -> negate_dsp48/1
  opcode3/1 -> negate_dsp48/3
  alucode3/1 -> negate_dsp48/4
  carryin3/1 -> negate_dsp48/5
  carryinsel3/1 -> negate_dsp48/6
  Reinterpret/1 -> Convert1/1
  Convert1/1 -> Out1/1

== system fft_biplex_test3/fft_biplex_real_4x1/bi_real_unscr_4x/mirror_spectrum/complex_conj3/negate_dsp48 ==
  In1 : Inport
  Convert : xbsIndex_r4/Convert  arith_type="Signed  (2's comp)"  n_bits=18  bin_pt=input_bin_pt  quantization=Truncate  overflow=Wrap  en=off  latency=0  dbl_ovrd=off  pipeline=off  block_type=convert
      settings: block_version=11.4
  Convert1 : xbsIndex_r4/Convert  arith_type="Signed  (2's comp)"  n_bits=input_bit_width  bin_pt=input_bin_pt  quantization=Truncate  overflow=Wrap  en=off  latency=0  dbl_ovrd=off  pipeline=off  block_type=convert
      settings: block_version=11.4
  Reinterpret : xbsIndex_r4/Reinterpret  force_arith_type=on  arith_type="Signed  (2's comp)"  force_bin_pt=on  bin_pt=input_bin_pt  block_type=reinterpret
      settings: infoedit="Changes signal type without altering the binary representation.   You can changed the signal between signed and unsigned, and relocate the binary point.<br><br>Hardware notes: In hardware this block costs nothing.<br><br>Example:  Suppose the input is 6 bits wide, signed, with 2 fractional bits, and the output is forced to unsigned with 0 fractional bits.  Then an input of -2.0 (1110.00 in binary 2's complement) becomes an output of 56 (111000 in binary)."
  Reinterpret1 : xbsIndex_r4/Reinterpret  force_arith_type=on  arith_type="Signed  (2's comp)"  force_bin_pt=on  bin_pt=0  block_type=reinterpret
      settings: infoedit="Changes signal type without altering the binary representation.   You can changed the signal between signed and unsigned, and relocate the binary point.<br><br>Hardware notes: In hardware this block costs nothing.<br><br>Example:  Suppose the input is 6 bits wide, signed, with 2 fractional bits, and the output is forced to unsigned with 0 fractional bits.  Then an input of -2.0 (1110.00 in binary 2's complement) becomes an output of 56 (111000 in binary)."
  alucode3 : xbsIndex_r4/Constant  arith_type=Unsigned  const=0  n_bits=4  bin_pt=0  explicit_period=on  period=1  equ=P=C  opselect=C  inp2=PCIN>>17  opr=+  inp1=P  carry=CIN  dbl_ovrd=off  block_type=constant
  carryin3 : xbsIndex_r4/Constant  arith_type=Unsigned  const=0  n_bits=1  bin_pt=0  explicit_period=on  period=1  equ=P=C  opselect=C  inp2=PCIN>>17  opr=+  inp1=P  carry=CIN  dbl_ovrd=off  block_type=constant
  carryinsel3 : xbsIndex_r4/Constant  arith_type=Unsigned  const=0  n_bits=3  bin_pt=0  explicit_period=on  period=1  equ=P=C  opselect=C  inp2=PCIN>>17  opr=+  inp1=P  carry=CIN  dbl_ovrd=off  block_type=constant
  negate_dsp48 : xbsIndex_r4/DSP48E  use_a=Direct from A Port  use_b=Direct from B Port  reset_preg=off  pattern_from_creg=off  pattern='000000000000'  mask_from_creg=off  pattern_mask='3FFFFFFFFFFF'  sel_rounding_mask=Select mask  use_op=off  use_creg=off  rst_all=off  en_all=off  use_pcin=off  use_carrycascin=off  use_multsignin=off  use_carryout=off  use_patterndetect=off  use_patternbdetect=off  use_overflow=off  use_underflow=off  use_acout=off  use_bcout=off  use_pcout=off  use_multsignout=off  use_carrycascout=off  pipeline_a=1  pipeline_b=1  pipeline_acout=1  pipeline_bcout=1  pipeline_c=on  pipeline_p=on  pipeline_mult=on  pipeline_opmode=on  pipeline_alumode=on  pipeline_carryin=on  pipeline_carryinsel=on  rst_a=off  rst_b=off  rst_c=off  rst_mult=off  rst_p=off  rst_carry_in=off  rst_alumode=off  rst_ctrl=off  en_a1=off  en_a2=off  en_b1=off  en_b2=off  en_c=off  en_mult=off  en_p=off  en_carry_in=off  en_alumode=off  en_multcarryin=off  en_ctrl=off  use_synth_model=off  addsub_mode=ONE48  xl_useadderonly=off  block_type=dsp48e
      settings: block_version=10.1.3
  opcode1 : xbsIndex_r4/Constant  arith_type=Signed (2's comp)  const=-1  n_bits=30  bin_pt=0  explicit_period=on  period=1  equ=P=C  opselect=C  inp2=PCIN>>17  opr=+  inp1=P  carry=CIN  dbl_ovrd=off  block_type=constant
  opcode3 : xbsIndex_r4/Constant  arith_type=Unsigned  const=5  n_bits=7  bin_pt=0  explicit_period=on  period=1  equ=P=C  opselect=C  inp2=PCIN>>17  opr=+  inp1=P  carry=CIN  dbl_ovrd=off  block_type=constant
  Out1 : Outport
  wires:
  Convert1/1 -> Out1/1
  Reinterpret/1 -> Convert1/1
  carryinsel3/1 -> negate_dsp48/6
  carryin3/1 -> negate_dsp48/5
  alucode3/1 -> negate_dsp48/4
  opcode3/1 -> negate_dsp48/3
  opcode1/1 -> negate_dsp48/1
  Convert/1 -> Reinterpret1/1
  Reinterpret1/1 -> negate_dsp48/2
  In1/1 -> Convert/1
  negate_dsp48/1 -> Reinterpret/1

== system fft_biplex_test3/fft_biplex_real_4x1/biplex_core/fft_stage_1/butterfly_direct/convert_of1 ==
  din : Inport
  all_0s : xbsIndex_r4/Logical  logical_function=NAND  inputs=2  en=off  latency=latency  precision=Full  arith_type=Unsigned  n_bits=16  bin_pt=0  align_bp=on  dbl_ovrd=off  block_type=logical
  all_1s : xbsIndex_r4/Logical  logical_function=NAND  inputs=2  en=off  latency=latency  precision=Full  arith_type=Unsigned  n_bits=16  bin_pt=0  align_bp=on  dbl_ovrd=off  block_type=logical
  and : xbsIndex_r4/Logical  logical_function=AND  inputs=2  en=off  latency=0  precision=Full  arith_type=Unsigned  n_bits=16  bin_pt=0  align_bp=on  dbl_ovrd=off  block_type=logical
  convert : xbsIndex_r4/Convert  arith_type="Signed  (2's comp)"  n_bits=bit_width_o  bin_pt=binary_point_o  quantization=Truncate  overflow=Wrap  en=off  latency=latency  dbl_ovrd=off  pipeline=on  block_type=convert
      settings: block_version=10.1.1
  invert1 : xbsIndex_r4/Inverter  en=off  latency=0  dbl_ovrd=off  block_type=inv
  invert2 : xbsIndex_r4/Inverter  en=off  latency=0  dbl_ovrd=off  block_type=inv
  slice1 : xbsIndex_r4/Slice  nbits=1  boolean_output=on  mode=Upper Bit Location + Width  bit1=0  base1=MSB of Input  bit0=0  base0=LSB of Input  dbl_ovrd=off  block_type=slice
      settings: infoedit="Extracts a given range of bits from each input sample and presents it at the output.  The output type is ordinarily unsigned with binary point at zero, but can be Boolean when the slice is one bit wide.<P><P>Hardware notes: In hardware this block costs nothing."  block_version=10.1.3
  slice2 : xbsIndex_r4/Slice  nbits=1  boolean_output=on  mode=Upper Bit Location + Width  bit1=-1  base1=MSB of Input  bit0=0  base0=LSB of Input  dbl_ovrd=off  block_type=slice
      settings: infoedit="Extracts a given range of bits from each input sample and presents it at the output.  The output type is ordinarily unsigned with binary point at zero, but can be Boolean when the slice is one bit wide.<P><P>Hardware notes: In hardware this block costs nothing."  block_version=10.1.3
  dout : Outport
  of : Outport  Port=2
  wires:
  and/1 -> of/1
  all_1s/1 -> and/2
  all_0s/1 -> and/1
  invert2/1 -> all_0s/2
  slice2/1 -> invert2/1, all_1s/2
  invert1/1 -> all_0s/1
  slice1/1 -> invert1/1, all_1s/1
  convert/1 -> dout/1
  din/1 -> slice2/1, slice1/1, convert/1
